simulink model "Sterowanie_liniowe_obiektem_strukturalnie_niestabilnym"  (R2015a)
settings: Solver=ode3  StartTime=0.0  StopTime=30  FixedStep=0.001  RelTol=1e-3
values from neighbouring files (symbols this model uses):
  kd = 17    [Sterowanie_liniowe_obiektem_strukturalnie_niestabilnym.m]
  ki = 60    [Sterowanie_liniowe_obiektem_strukturalnie_niestabilnym.m]
  kp = 80    [Sterowanie_liniowe_obiektem_strukturalnie_niestabilnym.m]
undefined symbols (not defined in the file or in its folder): licz, licz2, mian, mian2, sigbuilder_block
settings Model: Creator=238  LastModifiedBy=238

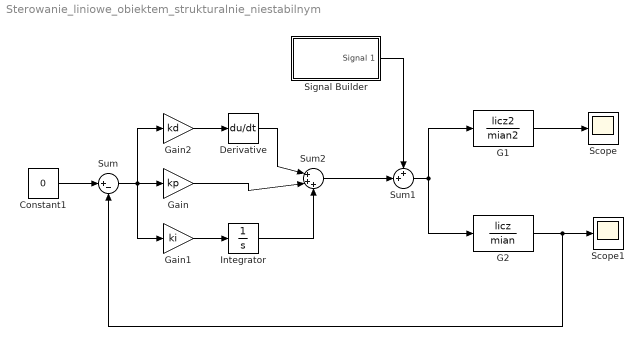
== system Sterowanie_liniowe_obiektem_strukturalnie_niestabilnym ==
  Constant1 : Constant  Value=0
  Derivative : Derivative
  G1 : TransferFcn  Numerator=licz2  Denominator=mian2
  G2 : TransferFcn  Numerator=licz  Denominator=mian
  Gain : Gain  Gain=kp
  Gain1 : Gain  Gain=ki
  Gain2 : Gain  Gain=kd
  Integrator : Integrator
  Scope : Scope
  Scope1 : Scope
  Signal Builder : Subsystem  Tag=STV Subsys  LoadFcn=sigbuilder_block('load');  StartFcn=sigbuilder_block('start');  StopFcn=sigbuilder_block('stop');  ClipboardFcn=sigbuilder_block('clipboard');  mask(Sigbuilder block){}
      mask help: Simulink:masks:SigbuilderBlock_MD
      mask init:
      | if ~strcmp(get_param(bdroot(gcbh),'SimulationStatus'),'stopped') tuvar = sigbuilder_block('maskInit'); end
      settings: CopyFcn=sigbuilder_block('copy');  DeleteFcn=sigbuilder_block('delete');  ModelCloseFcn=sigbuilder_block('modelClose');  PreSaveFcn=sigbuilder_block('preSave');  PauseFcn=sigbuilder_block('pause');  ContinueFcn=sigbuilder_block('continue');  NameChangeFcn=sigbuilder_block('namechange');  OpenFcn=sigbuilder_block('open',[437.6 199.2 550.4 400 ]);  CloseFcn=sigbuilder_block('close');
      mask Display: plot(0, 0, 100, 100,[2, 2, 32, 32, 2], [68, 8, 8, 68, 68],[32, 2], [38, 38], [32, 19, 2],[53, 60, 44], [32, 17, 17, 2],[16, 16, 31, 31]);txt = getActiveGroup(gcbh);text(2, 100, txt,'verticalAlignment', 'top');
  Sum : Sum  Inputs=|+-
  Sum1 : Sum  Inputs=++|
  Sum2 : Sum  Inputs=|+++
  wires:
  Constant1/1 -> Sum/1
  Sum1/1 -> G1/1, G2/1
  G2/1 -> Sum/2, Scope1/1
  G1/1 -> Scope/1
  Signal Builder/1(Signal 1) -> Sum1/1
  Sum/1 -> Gain1/1, Gain2/1, Gain/1
  Gain1/1 -> Integrator/1
  Gain2/1 -> Derivative/1
  Integrator/1 -> Sum2/3
  Gain/1 -> Sum2/2
  Derivative/1 -> Sum2/1
  Sum2/1 -> Sum1/2

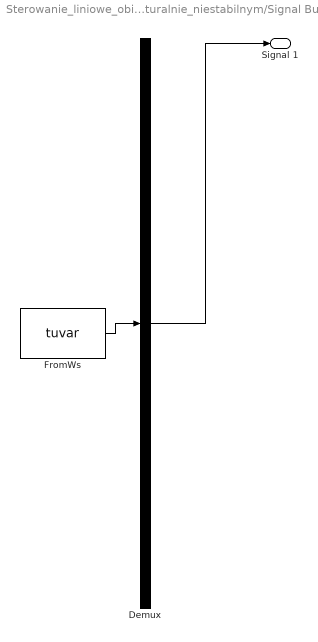
== system Sterowanie_liniowe_obiektem_strukturalnie_niestabilnym/Signal Builder ==
  Demux : Demux  Tag=STV Demux  Outputs=1
  FromWs : FromWorkspace  Tag=STV FromWs  VariableName=tuvar  SampleTime=0
      SigBuilderData=|
      | common.afterFinalStr = 'Extrapolate'
      | common.sampleTime = 0
      | dataSet.timeRange = [0 10]
      | dataSet.name = 'Group 1'
      | sbobj.Groups.Name = 'Group 1'
      | sbobj.Groups.Signals.Name = 'Signal 1'
      | sbobj.Groups.Signals.XData = [0 4 4 6 6 10]
      | sbobj.Groups.Signals.YData = [0 0 1 1 0 0]
  Signal 1 : Outport  Tag=STV Outport
  wires:
  Demux/1 -> Signal 1/1
  FromWs/1 -> Demux/1
